simulink library "nl_vehicle_MPC_lib"  (R2024b)
settings: Solver=VariableStepAuto  StartTime=0.0  StopTime=10.0  RelTol=1e-3
settings Model: Creator=tshintai  LastModifiedBy=tshintai
settings SolverCC: AlgebraicLoopSolver=TrustRegion
settings OptimizationCC: ReuseModelBlockBuffer=off
settings DebuggingCC: UnconnectedInputMsg=warning  UnconnectedOutputMsg=warning  UnconnectedLineMsg=warning
settings ModelReferenceCC: EnableRefExpFcnMdlSchedulingChecks=on
settings RTWCC: GPUComputeCapability=3.5  DLArmComputeVersion=19.05

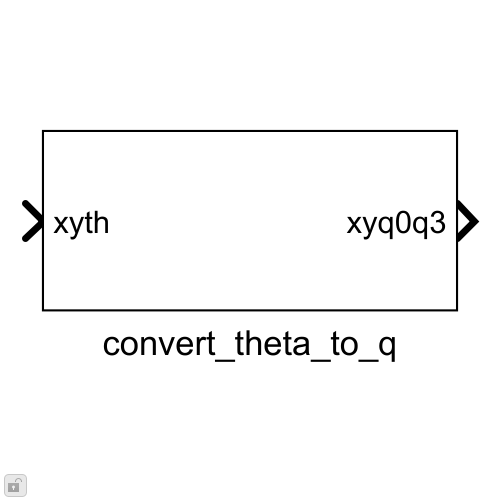
[thumbnail: Simulink's stored preview of the top-level diagram]
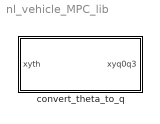
== system nl_vehicle_MPC_lib ==
  convert_theta_to_q : Subsystem

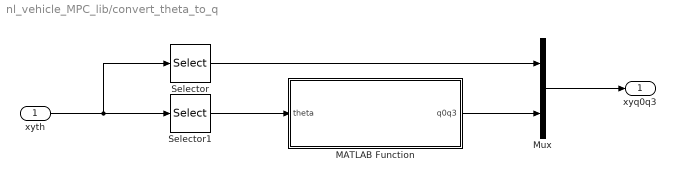
== system nl_vehicle_MPC_lib/convert_theta_to_q ==
  xyth : Inport
  MATLAB Function : MATLAB Function  TreatAsAtomicUnit=on
  Mux : Mux  Inputs=2
  Selector : Selector  InputPortWidth=3  IndexOptions=Index vector (dialog)  Indices=[1 2]  OutputSizes=1
  Selector1 : Selector  InputPortWidth=3  IndexOptions=Index vector (dialog)  Indices=[3]  OutputSizes=1
  xyq0q3 : Outport
  wires:
  MATLAB Function/1(q0q3) -> Mux/2
  Selector1/1 -> MATLAB Function/1(theta)
  xyth/1 -> Selector1/1, Selector/1
  Mux/1 -> xyq0q3/1
  Selector/1 -> Mux/1

== matlab function nl_vehicle_MPC_lib/convert_theta_to_q/MATLAB Function ==
  data: theta input; q0q3 output
function q0q3 = theta_to_q0q3_no_outlier(theta)

persistent initial_flag;
if isempty(initial_flag)
    initial_flag = false;
end
persistent q0q3_pre;
if isempty(q0q3_pre)
    q0q3_pre = zeros(2, 1, 'like', theta);
end

THETA = 0.5 * theta;
q0q3 = [cos(THETA); sin(THETA)];

if (~initial_flag)
    q0q3_pre = q0q3;
    initial_flag = true;
else
    diff = sum(abs(q0q3 - q0q3_pre));
        
    if (diff > 0.5)
        THETA_2 = 0.5 * (theta + 2 * pi);
        q0q3 = [cos(THETA_2); sin(THETA_2)];
        q0q3_pre = q0q3;
    else
        q0q3_pre = q0q3;
    end

end

end
